simulink model "prev_version"  (R2020b)
settings: Solver=VariableStepAuto  StartTime=0.0  StopTime=60  RelTol=1e-3
libraries: simulink x3
settings Model: Creator=PUGAZH  LastModifiedBy=PUGAZH
settings DebuggingCC: SFMachineParentedDataDiag=error

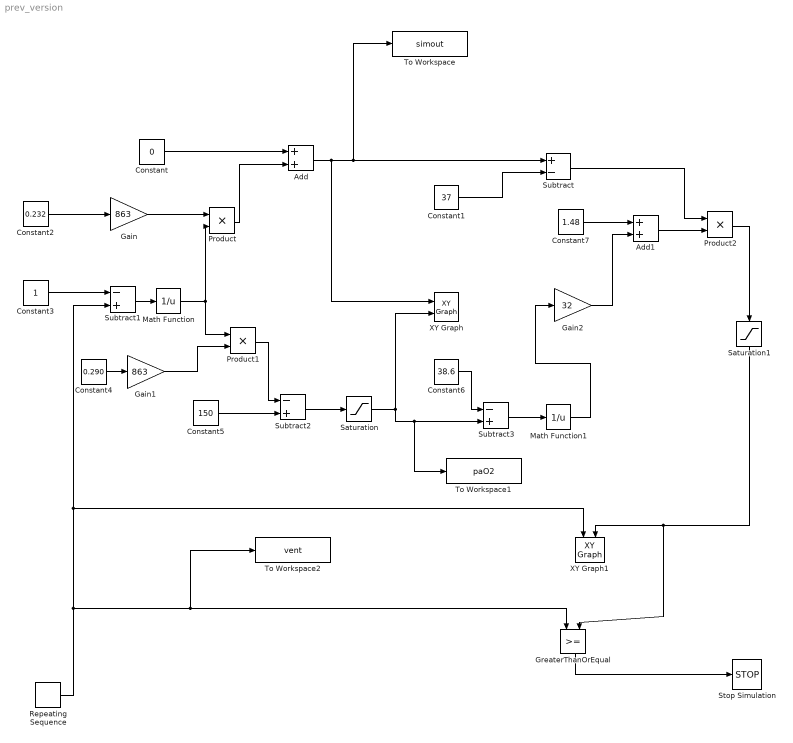
== system prev_version ==
  Add : Sum
  Add1 : Sum
  Constant : Constant  Value=0
  Constant1 : Constant  Value=37
  Constant2 : Constant  Value=0.232
  Constant3 : Constant
  Constant4 : Constant  Value=0.290
  Constant5 : Constant  Value=150
  Constant6 : Constant  Value=38.6
  Constant7 : Constant  Value=1.48
  Gain : Gain  Gain=863
  Gain1 : Gain  Gain=863
  Gain2 : Gain  Gain=32
  GreaterThanOrEqual : RelationalOperator  OutDataTypeStr=boolean  RndMeth=Simplest
  Math Function : Math  Operator=reciprocal  SaturateOnIntegerOverflow=on
  Math Function1 : Math  Operator=reciprocal  SaturateOnIntegerOverflow=on
  Product : Product
  Product1 : Product
  Product2 : Product
  Repeating Sequence : simulink/Sources/Repeating Sequence  rep_seq_t=[0 10]  rep_seq_y=[0 10]
  Saturation : Saturate
  Saturation1 : Saturate
  Stop Simulation : Stop
  Subtract : Sum  Inputs=+-
  Subtract1 : Sum  Inputs=-+
  Subtract2 : Sum  Inputs=-+
  Subtract3 : Sum  Inputs=-+
  To Workspace : ToWorkspace  VariableName=simout  SaveFormat=Timeseries  SampleTime=-1
  To Workspace1 : ToWorkspace  VariableName=paO2  SaveFormat=Timeseries  SampleTime=-1
      settings: Decimation=100
  To Workspace2 : ToWorkspace  VariableName=vent  SaveFormat=Timeseries  SampleTime=-1
  XY Graph : simulink/Sinks/XY Graph  xmin=-1  xmax=1  ymin=-1  ymax=1  st=-1
  XY Graph1 : simulink/Sinks/XY Graph  xmin=-1  xmax=1  ymin=-1  ymax=1  st=-1
  wires:
  Add/1 -> XY Graph/1, Subtract/1, To Workspace/1
  Product/1 -> Add/2
  Gain/1 -> Product/1
  Constant1/1 -> Subtract/2
  Constant/1 -> Add/1
  Constant2/1 -> Gain/1
  Constant3/1 -> Subtract1/1
  Subtract1/1 -> Math Function/1
  Math Function/1 -> Product/2, Product1/1
  Constant4/1 -> Gain1/1
  Gain1/1 -> Product1/2
  Constant5/1 -> Subtract2/2
  Product1/1 -> Subtract2/1
  Subtract2/1 -> Saturation/1
  Saturation/1 -> XY Graph/2, To Workspace1/1, Subtract3/2
  Constant6/1 -> Subtract3/1
  Subtract3/1 -> Math Function1/1
  Math Function1/1 -> Gain2/1
  Gain2/1 -> Add1/2
  Constant7/1 -> Add1/1
  Subtract/1 -> Product2/1
  Add1/1 -> Product2/2
  Product2/1 -> Saturation1/1
  Saturation1/1 -> XY Graph1/2, GreaterThanOrEqual/2
  GreaterThanOrEqual/1 -> Stop Simulation/1
  Repeating Sequence/1 -> To Workspace2/1, GreaterThanOrEqual/1, XY Graph1/1, Subtract1/2
